simulink model "nonlinear_discrete_ADRC"  (R2018a)
settings: Solver=FixedStepAuto  StartTime=0.0  StopTime=100  FixedStep=0.1  RelTol=1e-3
InitFcn:
  | T = 0.1;
  | r = 30;
  | h = 0.1;
  | alpha1 = 0.5;
  | alpha2 = 0.5;
  | b = 1;
  | kp = 1.5;
  | kd = 4.5;
  | beta = [70 60 100];
settings Model: Creator=leony  LastModifiedBy=leony
settings SolverCC: ZeroCrossAlgorithm=Adaptive
settings DebuggingCC: MaxConsecutiveZCsMsg=none  IgnoredZcDiagnostic=none

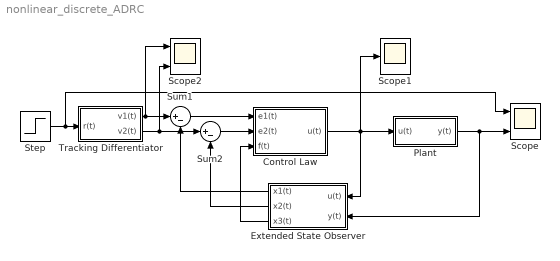
== system nonlinear_discrete_ADRC ==
  Control Law : Subsystem
  Extended State Observer : Subsystem
  Plant : Subsystem
  Scope : Scope  NumInputPorts=2
  Scope1 : Scope
  Scope2 : Scope  NumInputPorts=2
  Step : Step  SampleTime=0
  Sum1 : Sum  Inputs=|+-
  Sum2 : Sum  Inputs=|+-
  Tracking Differentiator : Subsystem
  wires:
  Tracking Differentiator/1(v1(t)) -> Scope2/1, Sum1/1
  Extended State Observer/1(x1(t)) -> Sum1/2
  Tracking Differentiator/2(v2(t)) -> Scope2/2, Sum2/1
  Extended State Observer/2(x2(t)) -> Sum2/2
  Sum1/1 -> Control Law/1(e1(t))
  Sum2/1 -> Control Law/2(e2(t))
  Extended State Observer/3(x3(t)) -> Control Law/3(f(t))
  Control Law/1(u(t)) -> Scope1/1, Plant/1(u(t)), Extended State Observer/1(u(t))
  Plant/1(y(t)) -> Scope/2, Extended State Observer/2(y(t))
  Step/1 -> Scope/1, Tracking Differentiator/1(r(t))

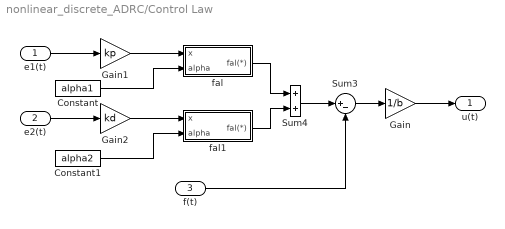
== system nonlinear_discrete_ADRC/Control Law ==
  e1(t) : Inport
  e2(t) : Inport  Port=2
  f(t) : Inport  Port=3
  Constant : Constant  Value=alpha1
  Constant1 : Constant  Value=alpha2
  Gain : Gain  Gain=1/b
  Gain1 : Gain  Gain=kp
  Gain2 : Gain  Gain=kd
  Sum3 : Sum  Inputs=|+-
  Sum4 : Sum
  fal : Subsystem
  fal1 : Subsystem
  u(t) : Outport
  wires:
  Sum3/1 -> Gain/1
  fal1/1(fal(*)) -> Sum4/2
  Constant1/1 -> fal1/2(alpha)
  Constant/1 -> fal/2(alpha)
  fal/1(fal(*)) -> Sum4/1
  Sum4/1 -> Sum3/1
  Gain/1 -> u(t)/1
  f(t)/1 -> Sum3/2
  Gain1/1 -> fal/1(x)
  e1(t)/1 -> Gain1/1
  Gain2/1 -> fal1/1(x)
  e2(t)/1 -> Gain2/1

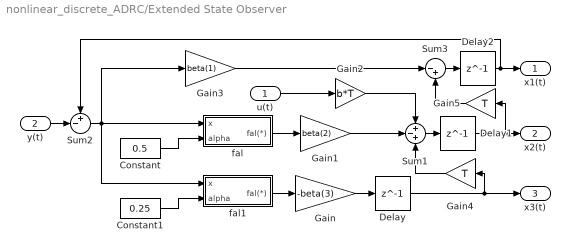
== system nonlinear_discrete_ADRC/Extended State Observer ==
  u(t) : Inport
  y(t) : Inport  Port=2
  Constant : Constant  Value=0.5
  Constant1 : Constant  Value=0.25
  Delay : Delay  DelayLength=1  InitialCondition=0
  Delay1 : Delay  DelayLength=1  InitialCondition=0
  Delay2 : Delay  DelayLength=1  InitialCondition=0
  Gain : Gain  Gain=-beta(3)
  Gain1 : Gain  Gain=beta(2)
  Gain2 : Gain  Gain=b*T
  Gain3 : Gain  Gain=beta(1)
  Gain4 : Gain  Gain=T
  Gain5 : Gain  Gain=T
  Sum1 : Sum  Inputs=+-+
  Sum2 : Sum  Inputs=+-|
  Sum3 : Sum  Inputs=|-+
  fal : Subsystem
  fal1 : Subsystem
  x1(t) : Outport
  x2(t) : Outport  Port=2
  x3(t) : Outport  Port=3
  wires:
  fal1/1(fal(*)) -> Gain/1
  fal/1(fal(*)) -> Gain1/1
  Constant1/1 -> fal1/2(alpha)
  Delay2/1 -> Sum2/1, x1(t)/1
  Sum1/1 -> Delay1/1
  Gain/1 -> Delay/1
  Delay/1 -> Gain4/1, x3(t)/1
  Gain1/1 -> Sum1/2
  Delay1/1 -> Gain5/1, x2(t)/1
  Sum2/1 -> Gain3/1, fal/1(x), fal1/1(x)
  Constant/1 -> fal/2(alpha)
  Sum3/1 -> Delay2/1
  y(t)/1 -> Sum2/2
  u(t)/1 -> Gain2/1
  Gain2/1 -> Sum1/1
  Gain3/1 -> Sum3/1
  Gain4/1 -> Sum1/3
  Gain5/1 -> Sum3/2

== system nonlinear_discrete_ADRC/Plant ==
  u(t) : Inport
  Gain : Gain  Gain=6
  Gain1 : Gain
  Gain2 : Gain  Gain=9
  Integrator : Integrator
  Integrator1 : Integrator
  Sum : Sum  Inputs=--+||
  y(t) : Outport
  wires:
  Integrator/1 -> Gain/1, Integrator1/1
  Integrator1/1 -> Gain1/1, y(t)/1
  Sum/1 -> Integrator/1
  Gain/1 -> Sum/1
  Gain1/1 -> Sum/2
  Gain2/1 -> Sum/3
  u(t)/1 -> Gain2/1

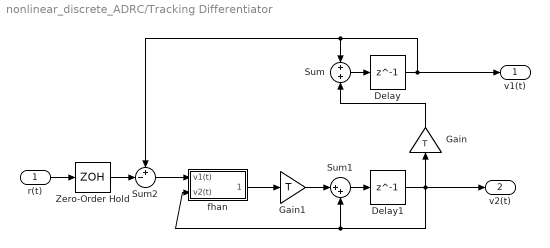
== system nonlinear_discrete_ADRC/Tracking Differentiator ==
  r(t) : Inport
  Delay : Delay  DelayLength=1  InitialCondition=0
  Delay1 : Delay  DelayLength=1  InitialCondition=0
  Gain : Gain  Gain=T
  Gain1 : Gain  Gain=T
  Sum : Sum
  Sum1 : Sum  Inputs=|++
  Sum2 : Sum  Inputs=+-|
  Zero-Order Hold : ZeroOrderHold  SampleTime=T
  fhan : Subsystem
  v1(t) : Outport
  v2(t) : Outport  Port=2
  wires:
  Gain/1 -> Sum/2
  Delay/1 -> Sum2/1, Sum/1, v1(t)/1
  Delay1/1 -> Gain/1, v2(t)/1, fhan/2(v2(t)), Sum1/2
  Sum/1 -> Delay/1
  Sum1/1 -> Delay1/1
  Sum2/1 -> fhan/1(v1(t))
  r(t)/1 -> Zero-Order Hold/1
  Zero-Order Hold/1 -> Sum2/2
  fhan/1(fhan(*)) -> Gain1/1
  Gain1/1 -> Sum1/1

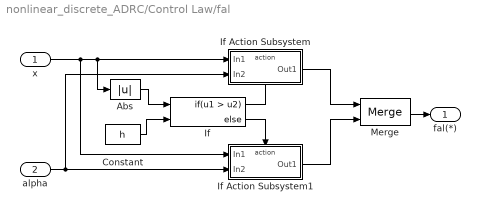
== system nonlinear_discrete_ADRC/Control Law/fal ==
  x : Inport
  alpha : Inport  Port=2
  Abs : Abs
  Constant : Constant  Value=h
  If : If  NumInputs=2  IfExpression=u1 > u2
  If Action Subsystem : Subsystem  TreatAsAtomicUnit=on
  If Action Subsystem1 : Subsystem  TreatAsAtomicUnit=on
  Merge : Merge
  fal(*) : Outport
  wires:
  x/1 -> If Action Subsystem1/1(In1), Abs/1, If Action Subsystem/1(In1)
  If/1 -> If Action Subsystem/Action
  If Action Subsystem1/1(Out1) -> Merge/2
  Abs/1 -> If/1
  Merge/1 -> fal(*)/1
  Constant/1 -> If/2
  If/2 -> If Action Subsystem1/Action
  If Action Subsystem/1(Out1) -> Merge/1
  alpha/1 -> If Action Subsystem/2(In2), If Action Subsystem1/2(In2)

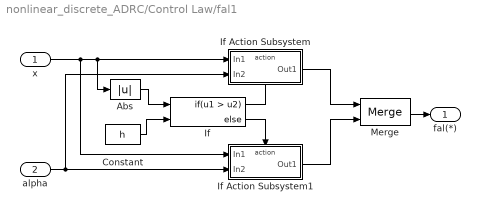
== system nonlinear_discrete_ADRC/Control Law/fal1 ==
  x : Inport
  alpha : Inport  Port=2
  Abs : Abs
  Constant : Constant  Value=h
  If : If  NumInputs=2  IfExpression=u1 > u2
  If Action Subsystem : Subsystem  TreatAsAtomicUnit=on
  If Action Subsystem1 : Subsystem  TreatAsAtomicUnit=on
  Merge : Merge
  fal(*) : Outport
  wires:
  x/1 -> If Action Subsystem1/1(In1), Abs/1, If Action Subsystem/1(In1)
  If/1 -> If Action Subsystem/Action
  If Action Subsystem1/1(Out1) -> Merge/2
  Abs/1 -> If/1
  Merge/1 -> fal(*)/1
  Constant/1 -> If/2
  If/2 -> If Action Subsystem1/Action
  If Action Subsystem/1(Out1) -> Merge/1
  alpha/1 -> If Action Subsystem/2(In2), If Action Subsystem1/2(In2)

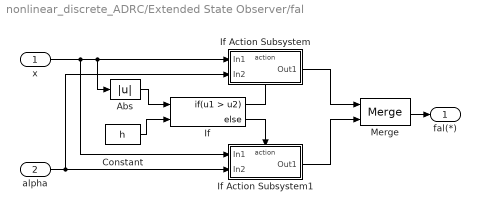
== system nonlinear_discrete_ADRC/Extended State Observer/fal ==
  x : Inport
  alpha : Inport  Port=2
  Abs : Abs
  Constant : Constant  Value=h
  If : If  NumInputs=2  IfExpression=u1 > u2
  If Action Subsystem : Subsystem  TreatAsAtomicUnit=on
  If Action Subsystem1 : Subsystem  TreatAsAtomicUnit=on
  Merge : Merge
  fal(*) : Outport
  wires:
  x/1 -> If Action Subsystem1/1(In1), Abs/1, If Action Subsystem/1(In1)
  If/1 -> If Action Subsystem/Action
  If Action Subsystem1/1(Out1) -> Merge/2
  Abs/1 -> If/1
  Merge/1 -> fal(*)/1
  Constant/1 -> If/2
  If/2 -> If Action Subsystem1/Action
  If Action Subsystem/1(Out1) -> Merge/1
  alpha/1 -> If Action Subsystem/2(In2), If Action Subsystem1/2(In2)

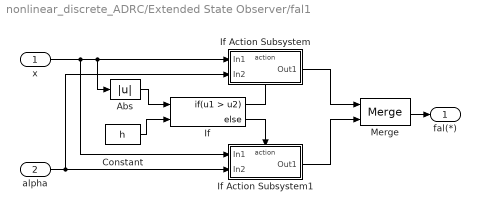
== system nonlinear_discrete_ADRC/Extended State Observer/fal1 ==
  x : Inport
  alpha : Inport  Port=2
  Abs : Abs
  Constant : Constant  Value=h
  If : If  NumInputs=2  IfExpression=u1 > u2
  If Action Subsystem : Subsystem  TreatAsAtomicUnit=on
  If Action Subsystem1 : Subsystem  TreatAsAtomicUnit=on
  Merge : Merge
  fal(*) : Outport
  wires:
  x/1 -> If Action Subsystem1/1(In1), Abs/1, If Action Subsystem/1(In1)
  If/1 -> If Action Subsystem/Action
  If Action Subsystem1/1(Out1) -> Merge/2
  Abs/1 -> If/1
  Merge/1 -> fal(*)/1
  Constant/1 -> If/2
  If/2 -> If Action Subsystem1/Action
  If Action Subsystem/1(Out1) -> Merge/1
  alpha/1 -> If Action Subsystem/2(In2), If Action Subsystem1/2(In2)

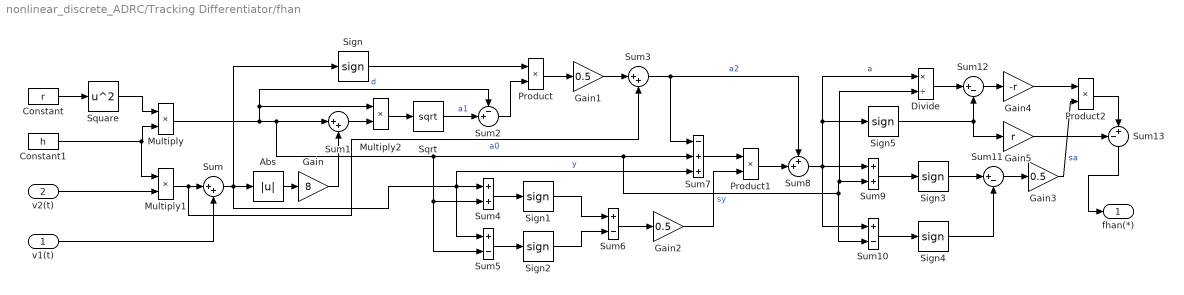
== system nonlinear_discrete_ADRC/Tracking Differentiator/fhan ==
  v1(t) : Inport
  v2(t) : Inport  Port=2
  Abs : Abs
  Constant : Constant  Value=r
  Constant1 : Constant  Value=h
  Divide : Product  Inputs=*/
  Gain : Gain  Gain=8
  Gain1 : Gain  Gain=0.5
  Gain2 : Gain  Gain=0.5
  Gain3 : Gain  Gain=0.5
  Gain4 : Gain  Gain=-r
  Gain5 : Gain  Gain=r
  Multiply : Product
  Multiply1 : Product
  Multiply2 : Product
  Product : Product
  Product1 : Product
  Product2 : Product
  Sign{,1..5} (6 alike) : Signum
  Sqrt : Sqrt  SaturateOnIntegerOverflow=on
  Square : Math  Operator=square  SaturateOnIntegerOverflow=on
  Sum : Sum  Inputs=|++
  Sum1 : Sum  Inputs=|++
  Sum10 : Sum  Inputs=+-
  Sum11 : Sum  Inputs=|+-
  Sum12 : Sum  Inputs=|+-
  Sum13 : Sum  Inputs=-+|
  Sum2 : Sum  Inputs=-+|
  Sum3 : Sum  Inputs=|++
  Sum4 : Sum
  Sum5 : Sum  Inputs=+-
  Sum6 : Sum  Inputs=+-
  Sum7 : Sum  Inputs=-++
  Sum8 : Sum  Inputs=++|
  Sum9 : Sum
  fhan(*) : Outport
  wires:
  Constant/1 -> Square/1
  Square/1 -> Multiply/1
  Constant1/1 -> Multiply1/1, Multiply/2
  v2(t)/1 -> Multiply1/2
  v1(t)/1 -> Sum/2
  Multiply1/1 -> Sum3/2, Sum/1  "a0"
  Multiply/1 -> Sum2/1, Multiply2/1, Sum5/2, Sum4/2, Sum10/2, Divide/2, Sum9/2, Sum7/2, Sum1/1  "d"
  Abs/1 -> Gain/1
  Sum/1 -> Sum7/3, Sum5/1, Sum4/1, Sign/1, Abs/1  "y"
  Gain/1 -> Sum1/2
  Sum1/1 -> Multiply2/2
  Multiply2/1 -> Sqrt/1
  Sign/1 -> Product/1
  Sqrt/1 -> Sum2/2  "a1"
  Sum2/1 -> Product/2
  Product/1 -> Gain1/1
  Gain1/1 -> Sum3/1
  Sum3/1 -> Sum8/1, Sum7/1  "a2"
  Sum4/1 -> Sign1/1
  Sum5/1 -> Sign2/1
  Sign1/1 -> Sum6/1
  Sign2/1 -> Sum6/2
  Sum6/1 -> Gain2/1
  Gain2/1 -> Product1/2  "sy"
  Sum7/1 -> Product1/1
  Product1/1 -> Sum8/2
  Sum8/1 -> Divide/1, Sign5/1, Sum10/1, Sum9/1  "a"
  Sum9/1 -> Sign3/1
  Sum10/1 -> Sign4/1
  Sign3/1 -> Sum11/1
  Sign4/1 -> Sum11/2
  Sum11/1 -> Gain3/1
  Gain3/1 -> Product2/2  "sa"
  Divide/1 -> Sum12/1
  Sign5/1 -> Gain5/1, Sum12/2
  Sum12/1 -> Gain4/1
  Gain4/1 -> Product2/1
  Gain5/1 -> Sum13/1
  Product2/1 -> Sum13/2
  Sum13/1 -> fhan(*)/1

== system nonlinear_discrete_ADRC/Control Law/fal/If Action Subsystem ==
  In1 : Inport
  In2 : Inport  Port=2
  Action Port : ActionPort  PropagateVarSize=During execution  ActionType=then
  Abs : Abs
  Power : Math  Operator=pow  SaturateOnIntegerOverflow=on
  Product : Product
  Sign : Signum
  Out1 : Outport
  wires:
  Abs/1 -> Power/1
  In2/1 -> Power/2
  In1/1 -> Sign/1, Abs/1
  Sign/1 -> Product/1
  Power/1 -> Product/2
  Product/1 -> Out1/1

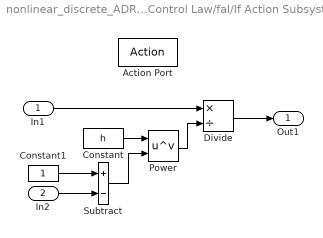
== system nonlinear_discrete_ADRC/Control Law/fal/If Action Subsystem1 ==
  In1 : Inport
  In2 : Inport  Port=2
  Action Port : ActionPort  PropagateVarSize=During execution  ActionType=else
  Constant : Constant  Value=h
  Constant1 : Constant
  Divide : Product  Inputs=*/
  Power : Math  Operator=pow  SaturateOnIntegerOverflow=on
  Subtract : Sum  Inputs=+-
  Out1 : Outport
  wires:
  In1/1 -> Divide/1
  Divide/1 -> Out1/1
  Constant/1 -> Power/1
  Constant1/1 -> Subtract/1
  In2/1 -> Subtract/2
  Subtract/1 -> Power/2
  Power/1 -> Divide/2

== system nonlinear_discrete_ADRC/Control Law/fal1/If Action Subsystem ==
  In1 : Inport
  In2 : Inport  Port=2
  Action Port : ActionPort  PropagateVarSize=During execution  ActionType=then
  Abs : Abs
  Power : Math  Operator=pow  SaturateOnIntegerOverflow=on
  Product : Product
  Sign : Signum
  Out1 : Outport
  wires:
  Abs/1 -> Power/1
  In2/1 -> Power/2
  In1/1 -> Sign/1, Abs/1
  Sign/1 -> Product/1
  Power/1 -> Product/2
  Product/1 -> Out1/1

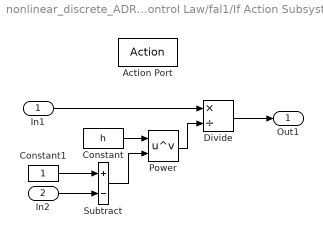
== system nonlinear_discrete_ADRC/Control Law/fal1/If Action Subsystem1 ==
  In1 : Inport
  In2 : Inport  Port=2
  Action Port : ActionPort  PropagateVarSize=During execution  ActionType=else
  Constant : Constant  Value=h
  Constant1 : Constant
  Divide : Product  Inputs=*/
  Power : Math  Operator=pow  SaturateOnIntegerOverflow=on
  Subtract : Sum  Inputs=+-
  Out1 : Outport
  wires:
  In1/1 -> Divide/1
  Divide/1 -> Out1/1
  Constant/1 -> Power/1
  Constant1/1 -> Subtract/1
  In2/1 -> Subtract/2
  Subtract/1 -> Power/2
  Power/1 -> Divide/2

== system nonlinear_discrete_ADRC/Extended State Observer/fal/If Action Subsystem ==
  In1 : Inport
  In2 : Inport  Port=2
  Action Port : ActionPort  PropagateVarSize=During execution  ActionType=then
  Abs : Abs
  Power : Math  Operator=pow  SaturateOnIntegerOverflow=on
  Product : Product
  Sign : Signum
  Out1 : Outport
  wires:
  Abs/1 -> Power/1
  In2/1 -> Power/2
  In1/1 -> Sign/1, Abs/1
  Sign/1 -> Product/1
  Power/1 -> Product/2
  Product/1 -> Out1/1

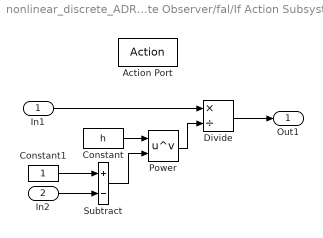
== system nonlinear_discrete_ADRC/Extended State Observer/fal/If Action Subsystem1 ==
  In1 : Inport
  In2 : Inport  Port=2
  Action Port : ActionPort  PropagateVarSize=During execution  ActionType=else
  Constant : Constant  Value=h
  Constant1 : Constant
  Divide : Product  Inputs=*/
  Power : Math  Operator=pow  SaturateOnIntegerOverflow=on
  Subtract : Sum  Inputs=+-
  Out1 : Outport
  wires:
  In1/1 -> Divide/1
  Divide/1 -> Out1/1
  Constant/1 -> Power/1
  Constant1/1 -> Subtract/1
  In2/1 -> Subtract/2
  Subtract/1 -> Power/2
  Power/1 -> Divide/2

== system nonlinear_discrete_ADRC/Extended State Observer/fal1/If Action Subsystem ==
  In1 : Inport
  In2 : Inport  Port=2
  Action Port : ActionPort  PropagateVarSize=During execution  ActionType=then
  Abs : Abs
  Power : Math  Operator=pow  SaturateOnIntegerOverflow=on
  Product : Product
  Sign : Signum
  Out1 : Outport
  wires:
  Abs/1 -> Power/1
  In2/1 -> Power/2
  In1/1 -> Sign/1, Abs/1
  Sign/1 -> Product/1
  Power/1 -> Product/2
  Product/1 -> Out1/1

== system nonlinear_discrete_ADRC/Extended State Observer/fal1/If Action Subsystem1 ==
  In1 : Inport
  In2 : Inport  Port=2
  Action Port : ActionPort  PropagateVarSize=During execution  ActionType=else
  Constant : Constant  Value=h
  Constant1 : Constant
  Divide : Product  Inputs=*/
  Power : Math  Operator=pow  SaturateOnIntegerOverflow=on
  Subtract : Sum  Inputs=+-
  Out1 : Outport
  wires:
  In1/1 -> Divide/1
  Divide/1 -> Out1/1
  Constant/1 -> Power/1
  Constant1/1 -> Subtract/1
  In2/1 -> Subtract/2
  Subtract/1 -> Power/2
  Power/1 -> Divide/2
